simulink model "pv_cell_model"  (Simulink 8.7)
settings: Solver=ode45  StartTime=0.0  StopTime=1  MaxStep=0.02  RelTol=1e-3
libraries: simulink x3
settings Model: Creator=motahhir  LastModifiedBy=Motahhir
settings DataIOCC: SignalLoggingSaveFormat=ModelDataLogs
settings OptimizationCC: ExpressionDepthLimit=2147483647
settings DebuggingCC: SolverPrmCheckMsg=warning  FcnCallInpInsideContextMsg=EnableAllAsWarning  StateNameClashWarn=warning
settings ConfigComp: CovSFcnEnable=off

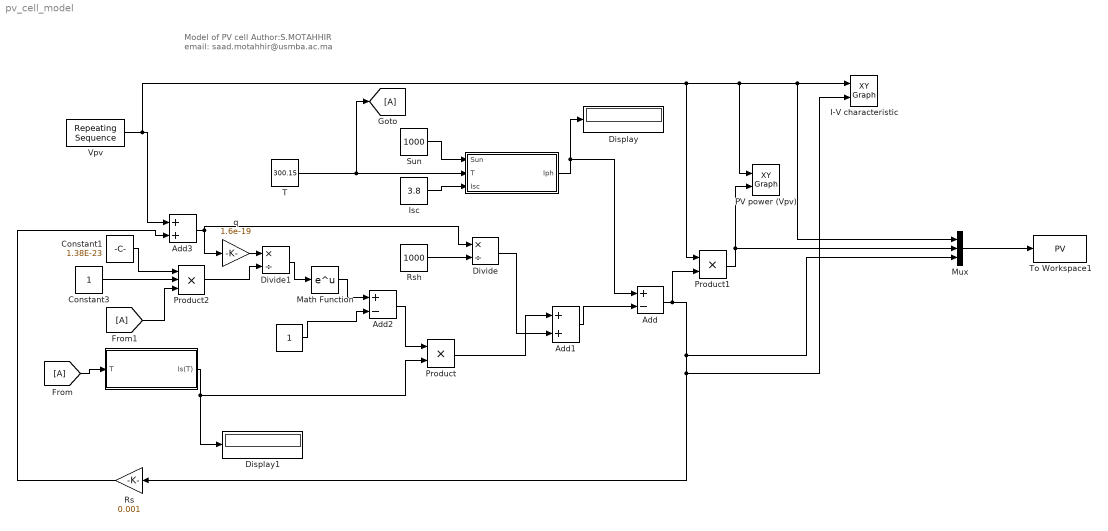
== system pv_cell_model ==
  note: Model of PV cell
      | Author:S.MOTAHHIR
      | email: saad.motahhir@usmba.ac.ma
  " " : Subsystem
  "  " : Constant
  "                         " : Subsystem
      mask init:
      | q=1.6e-19;
      | T=300.15; 
      | Tnom=300.15;
      | K=1.38e-23;
      | N=1.5;
      | vt=T*K/q;
      | Is=1e-9;
      | Eg=1.12;
  Add : Sum  Inputs=+-
  Add1 : Sum
  Add2 : Sum  Inputs=+-
  Add3 : Sum
  Constant1 : Constant  Value=1.38E-23
  Constant3 : Constant
  Display : Display
  Display1 : Display
  Divide : Product  Inputs=*/
  Divide1 : Product  Inputs=*/
  I-V characteristic : simulink/Sinks/XY Graph  xmin=0  xmax=0.7  ymin=0  ymax=4  st=-1
  Isc : Constant  Value=3.8
  Math Function : Math  SaturateOnIntegerOverflow=on
  Mux : Mux  Inputs=3
  PV power (Vpv) : simulink/Sinks/XY Graph  xmin=0  xmax=0.7  ymin=0  ymax=2  st=-1
  Product : Product  RndMeth=Zero
  Product1 : Product  RndMeth=Zero
  Product2 : Product  Inputs=3  RndMeth=Zero
  Rs : Gain  Gain=0.001
  Rsh : Constant  Value=1000
  Sun : Constant  Value=1000
  T : Constant  Value=300.15
  To Workspace1 : ToWorkspace  VariableName=PV  SaveFormat=Structure With Time  SampleTime=-1
  Vpv : simulink/Sources/Repeating Sequence  rep_seq_t=[0 1 2]  rep_seq_y="[-0.1  0.6 -0.1]"
  q : Gain  Gain=1.6e-19
  wires:
  Sun/1 -> " "/1(Sun)
  Isc/1 -> " "/3(Isc)
  T/1 -> " "/2(T), [A]
  " "/1(Iph) -> Display/1, Add/1
  [A] -> "                         "/1(T)
  Divide/1 -> Add1/2
  Rsh/1 -> Divide/2
  "                         "/1(Is(T)) -> Product/2, Display1/1
  Add2/1 -> Product/1
  Math Function/1 -> Add2/1
  "  "/1 -> Add2/2
  Divide1/1 -> Math Function/1
  Add/1 -> Product1/2, Rs/1, I-V characteristic/2, Mux/3
  Product1/1 -> PV power (Vpv)/2, Mux/2
  Rs/1 -> Add3/2
  Product/1 -> Add1/1
  Add1/1 -> Add/2
  Vpv/1 -> Add3/1, PV power (Vpv)/1, I-V characteristic/1, Mux/1, Product1/1
  q/1 -> Divide1/1
  Add3/1 -> q/1, Divide/1
  Constant1/1 -> Product2/1
  [A] -> Product2/3
  Constant3/1 -> Product2/2
  Product2/1 -> Divide1/2
  Mux/1 -> To Workspace1/1

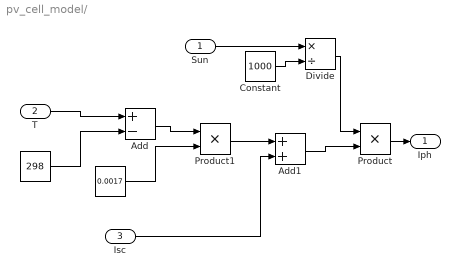
== system pv_cell_model/  ==
  Sun : Inport
  T : Inport  Port=2
  Isc : Inport  Port=3
  "   " : Constant  Value=298
  "                    " : Constant  Value=0.0017
  Add : Sum  Inputs=+-
  Add1 : Sum
  Constant : Constant  Value=1000
  Divide : Product  Inputs=*/
  Product : Product  RndMeth=Zero
  Product1 : Product  RndMeth=Zero
  Iph : Outport
  wires:
  Product/1 -> Iph/1
  Sun/1 -> Divide/1
  Constant/1 -> Divide/2
  T/1 -> Add/1
  "   "/1 -> Add/2
  Add/1 -> Product1/1
  "                    "/1 -> Product1/2
  Product1/1 -> Add1/1
  Add1/1 -> Product/2
  Isc/1 -> Add1/2
  Divide/1 -> Product/1

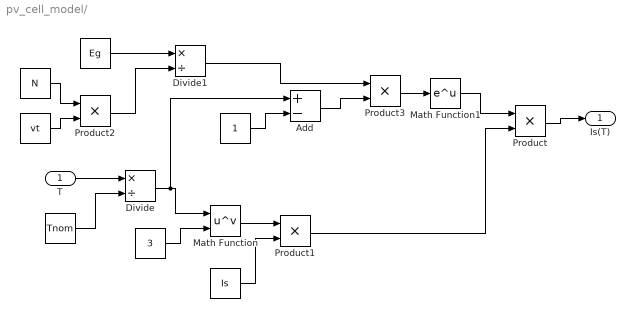
== system pv_cell_model/                          ==
  T : Inport
  " " : Constant
  "  " : Constant  Value=3
  "      " : Constant  Value=Is
  "        " : Constant  Value=Tnom
  "                      " : Constant  Value=Eg
  "                              " : Constant  Value=N
  "                               " : Constant  Value=vt
  Add : Sum  Inputs=+-
  Divide : Product  Inputs=*/
  Divide1 : Product  Inputs=*/
  Math Function : Math  Operator=pow  SaturateOnIntegerOverflow=on
  Math Function1 : Math  SaturateOnIntegerOverflow=on
  Product{,1..3} (4 alike) : Product  RndMeth=Zero
  Is(T) : Outport
  wires:
  Product/1 -> Is(T)/1
  T/1 -> Divide/1
  "        "/1 -> Divide/2
  Divide/1 -> Math Function/1, Add/1
  "  "/1 -> Math Function/2
  Math Function/1 -> Product1/1
  "      "/1 -> Product1/2
  Product1/1 -> Product/2
  "                               "/1 -> Product2/2
  "                              "/1 -> Product2/1
  Product2/1 -> Divide1/2
  "                      "/1 -> Divide1/1
  Math Function1/1 -> Product/1
  Product3/1 -> Math Function1/1
  Divide1/1 -> Product3/1
  Add/1 -> Product3/2
  " "/1 -> Add/2
